simulink model "newsimulation"  (R2015b)
settings: Solver=ode45  StartTime=0.0  StopTime=10  FixedStep=tsampling  RelTol=1e-3
values from neighbouring files (symbols this model uses):
  bHI = 35    [Initiation.m]
  bWall = 0    [Initiation.m]    (also in VirtualEnvironment.m = block.DialogPrm(2).Data; Virtual_Environment.m = block.DialogPrm(2).Data)
  kWall = 90000    [Initiation.m]    (also in VirtualEnvironment.m = block.DialogPrm(1).Data; Virtual_Environment.m = block.DialogPrm(1).Data)
  m = 1    [Initiation.m]
  nWall = 1    [Initiation.m]    (also in VirtualEnvironment.m = block.DialogPrm(3).Data; Virtual_Environment.m = block.DialogPrm(3).Data)
  tsampling = 0.001    [Initiation.m]    (also in VirtualEnvironment.m = block.DialogPrm(6).Data; Virtual_Environment.m = block.DialogPrm(6).Data)
  x0 = 0.14    [Initiation.m]    (also in PC.m = []; Wall.m = []; devision.m = []; sgn.m = [])
  x_dot0 = 0    [Initiation.m]
  xWall = 0.085    [Initiation.m]
libraries: simulink x4
settings Model: Creator=TOSHIBA  LastModifiedBy=TOSHIBA

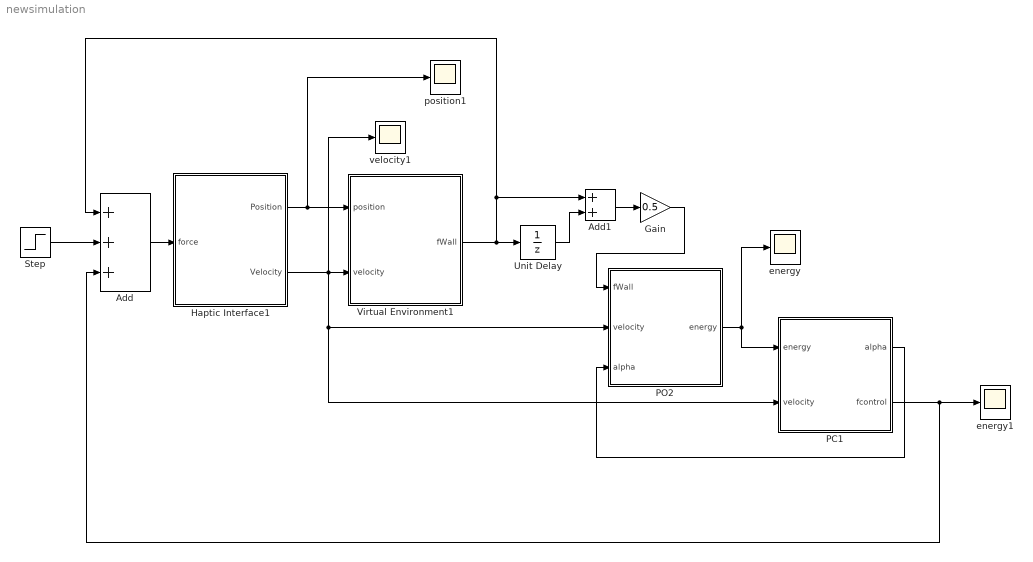
== system newsimulation ==
  Add : Sum  Inputs=+++
  Add1 : Sum
  Gain : Gain  Gain=0.5
  Haptic Interface1 : Subsystem
  PC1 : Subsystem
  PO2 : Subsystem
  Step : Step  Time=0.35  After=-10  SampleTime=0
  Unit Delay : UnitDelay  SampleTime=tsampling
  Virtual Environment1 : Subsystem
  energy : Scope
  energy1 : Scope
  position1 : Scope
  velocity1 : Scope
  wires:
  Haptic Interface1/1(Position) -> position1/1, Virtual Environment1/1(position)
  Add/1 -> Haptic Interface1/1(force)
  Step/1 -> Add/2
  Haptic Interface1/2(Velocity) -> PC1/2(velocity), PO2/2(velocity), Virtual Environment1/2(velocity), velocity1/1
  Virtual Environment1/1(fWall) -> Add1/1, Add/1, Unit Delay/1
  PO2/1(energy) -> PC1/1(energy), energy/1
  PC1/2(fcontrol) -> energy1/1, Add/3
  PC1/1(alpha) -> PO2/3(alpha)
  Add1/1 -> Gain/1
  Unit Delay/1 -> Add1/2
  Gain/1 -> PO2/1(fWall)

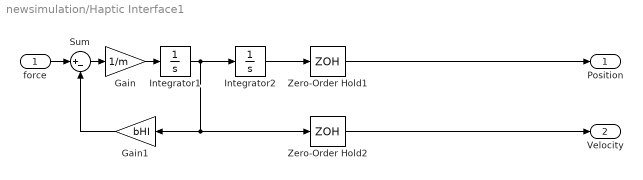
== system newsimulation/Haptic Interface1 ==
  force : Inport
  Gain : Gain  Gain=1/m
  Gain1 : Gain  Gain=bHI
  Integrator1 : Integrator  InitialCondition=x_dot0
  Integrator2 : Integrator  InitialCondition=x0
  Sum : Sum  Inputs=|+-
  Zero-Order Hold1 : ZeroOrderHold  SampleTime=tsampling
  Zero-Order Hold2 : ZeroOrderHold  SampleTime=tsampling
  Position : Outport
  Velocity : Outport  Port=2
  wires:
  Zero-Order Hold2/1 -> Velocity/1
  Integrator1/1 -> Zero-Order Hold2/1, Gain1/1, Integrator2/1
  Sum/1 -> Gain/1
  force/1 -> Sum/1
  Gain/1 -> Integrator1/1
  Gain1/1 -> Sum/2
  Integrator2/1 -> Zero-Order Hold1/1
  Zero-Order Hold1/1 -> Position/1

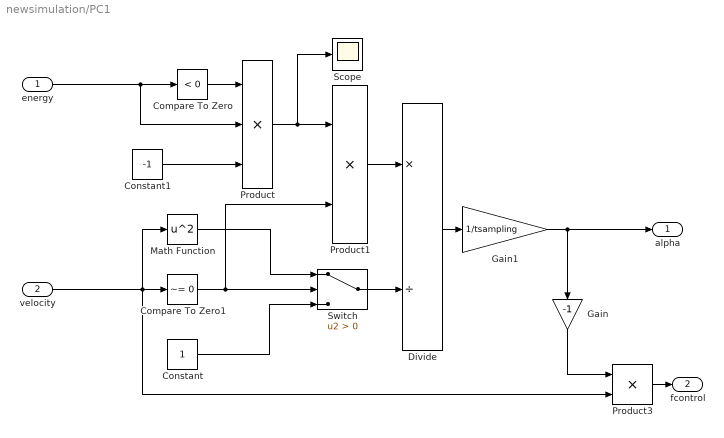
== system newsimulation/PC1 ==
  energy : Inport
  velocity : Inport  Port=2
  Compare To Zero : simulink/Logic and Bit Operations/Compare To Zero  relop=<  OutDataTypeStr=boolean
  Compare To Zero1 : simulink/Logic and Bit Operations/Compare To Zero  relop=~=  OutDataTypeStr=boolean
  Constant : Constant
  Constant1 : Constant  Value=-1
  Divide : Product  Inputs=*/
  Gain : Gain  Gain=-1
  Gain1 : Gain  Gain=1/tsampling
  Math Function : Math  Operator=square  SaturateOnIntegerOverflow=on
  Product : Product  Inputs=3
  Product1 : Product
  Product3 : Product
  Scope : Scope
  Switch : Switch  Criteria=u2 > Threshold
  alpha : Outport
  fcontrol : Outport  Port=2
  wires:
  Constant1/1 -> Product/3
  energy/1 -> Compare To Zero/1, Product/2
  Product/1 -> Product1/1, Scope/1
  Switch/1 -> Divide/2
  Gain1/1 -> alpha/1, Gain/1
  Product1/1 -> Divide/1
  Divide/1 -> Gain1/1
  Math Function/1 -> Switch/1
  Constant/1 -> Switch/3
  Compare To Zero1/1 -> Switch/2, Product1/2
  Compare To Zero/1 -> Product/1
  velocity/1 -> Compare To Zero1/1, Product3/2, Math Function/1
  Product3/1 -> fcontrol/1
  Gain/1 -> Product3/1

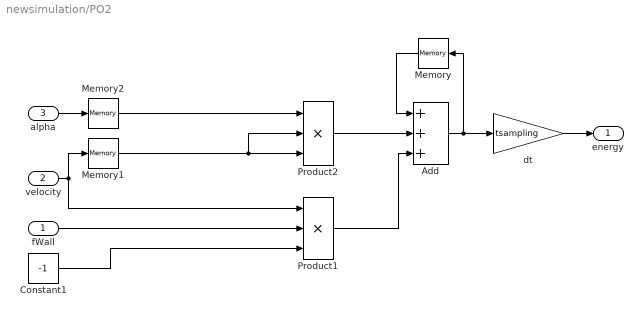
== system newsimulation/PO2 ==
  fWall : Inport
  velocity : Inport  Port=2
  alpha : Inport  Port=3
  Add : Sum  Inputs=+++
  Constant1 : Constant  Value=-1
  Memory : Memory
  Memory1 : Memory
  Memory2 : Memory
  Product1 : Product  Inputs=3
  Product2 : Product  Inputs=3
  dt : Gain  Gain=tsampling
  energy : Outport
  wires:
  velocity/1 -> Product1/1, Memory1/1
  fWall/1 -> Product1/2
  Product1/1 -> Add/3
  Constant1/1 -> Product1/3
  dt/1 -> energy/1
  Memory/1 -> Add/1
  Add/1 -> Memory/1, dt/1
  alpha/1 -> Memory2/1
  Product2/1 -> Add/2
  Memory2/1 -> Product2/1
  Memory1/1 -> Product2/2, Product2/3

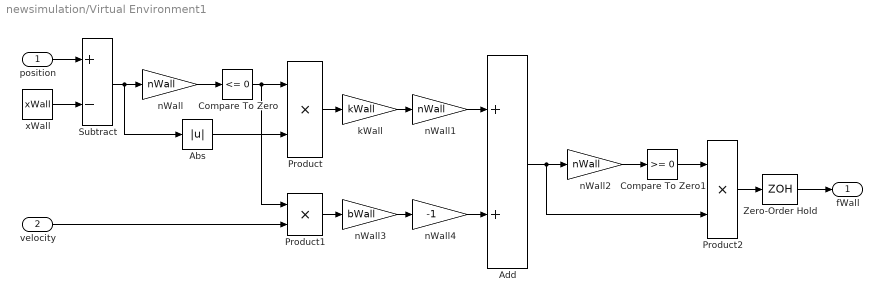
== system newsimulation/Virtual Environment1 ==
  position : Inport
  velocity : Inport  Port=2
  Abs : Abs
  Add : Sum
  Compare To Zero : simulink/Logic and Bit Operations/Compare To Zero  relop=<=  OutDataTypeStr=boolean
  Compare To Zero1 : simulink/Logic and Bit Operations/Compare To Zero  relop=>=  OutDataTypeStr=boolean
  Product : Product
  Product1 : Product
  Product2 : Product
  Subtract : Sum  Inputs=+-
  Zero-Order Hold : ZeroOrderHold  SampleTime=tsampling
  kWall : Gain  Gain=kWall
  nWall : Gain  Gain=nWall
  nWall1 : Gain  Gain=nWall
  nWall2 : Gain  Gain=nWall
  nWall3 : Gain  Gain=bWall
  nWall4 : Gain  Gain=-1
  xWall : Constant  Value=xWall
  fWall : Outport
  wires:
  Compare To Zero1/1 -> Product2/1
  nWall2/1 -> Compare To Zero1/1
  kWall/1 -> nWall1/1
  Product/1 -> kWall/1
  Abs/1 -> Product/2
  Compare To Zero/1 -> Product1/1, Product/1
  nWall/1 -> Compare To Zero/1
  Subtract/1 -> nWall/1, Abs/1
  position/1 -> Subtract/1
  xWall/1 -> Subtract/2
  nWall3/1 -> nWall4/1
  Product1/1 -> nWall3/1
  velocity/1 -> Product1/2
  nWall1/1 -> Add/1
  nWall4/1 -> Add/2
  Add/1 -> Product2/2, nWall2/1
  Product2/1 -> Zero-Order Hold/1
  Zero-Order Hold/1 -> fWall/1
